simulink model "modele_ericc_correcteur"  (R2016b)
settings: Solver=VariableStepAuto  StartTime=0.0  StopTime=2.5  RelTol=1e-3
InitFcn:
  | ericc3_DataFile
values from neighbouring files (symbols this model uses):
  Cr = 0.01    [data_modele_ericc.m]
  fv = 1/8547    (= 0.000117000117)    [data_modele_ericc.m]
  Jeq = fv*0.178    (= 2.0826020826e-05)    [data_modele_ericc.m]
  KAN = 2*1e6/1080    (= 1851.85185185)    [data_modele_ericc.m]
  Kc = 2000/(2*pi)    (= 318.309886184)    [data_modele_ericc.m]
  Kd = 0    [data_modele_ericc.m]
  Ki = 2E5    (= 200000)    [data_modele_ericc.m]
  Kp = 1e6    (= 1000000)    [data_modele_ericc.m]
  Kr = 3/1000    (= 0.003)    [data_modele_ericc.m]
  Ks = Kc/(Kr*KAN)    (= 57.2957795131)    [data_modele_ericc.m]
  Kt = 0.043    [data_modele_ericc.m]
  Kv = 0.17    [data_modele_ericc.m]
settings Model: Creator=emiliendurif  LastModifiedBy=emiliendurif
settings SolverCC: ZeroCrossAlgorithm=Adaptive

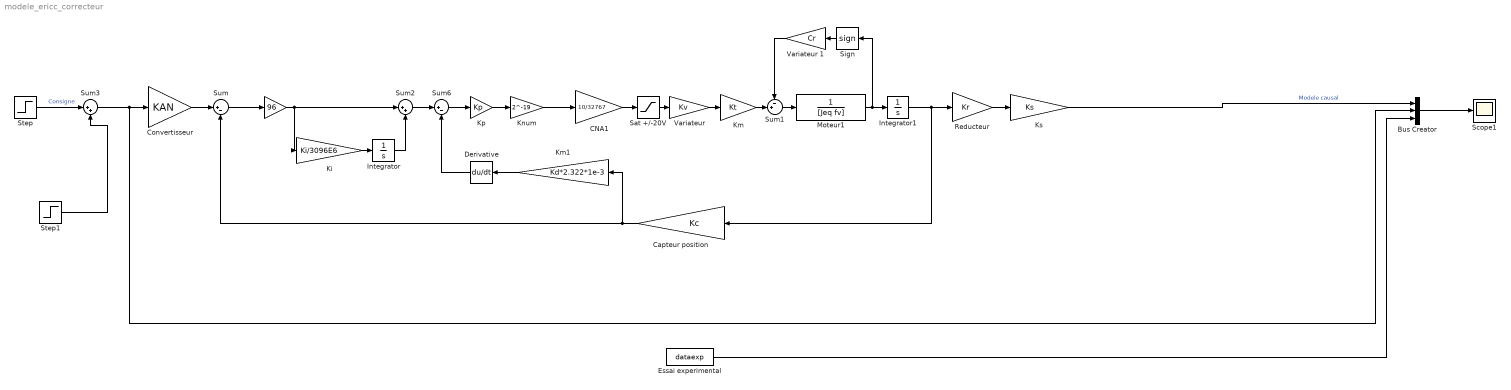
== system modele_ericc_correcteur ==
  " " : Gain  Gain=96
  Bus Creator : BusCreator  Inputs=3
  CNA1 : Gain  Gain=10/32767
  "Capteur position " : Gain  Gain=Kc
  Convertisseur : Gain  Gain=KAN
  Derivative : Derivative
  Essai experimental : FromWorkspace  VariableName=dataexp  OutDataTypeStr=fixdt('double', 'DataTypeOverride', 'Off')  SampleTime=0.007  OutputAfterFinalValue=Setting to zero
  Integrator : Integrator
  Integrator1 : Integrator
  Ki : Gain  Gain=Ki/3096E6
  Km : Gain  Gain=Kt
  Km1 : Gain  Gain=Kd*2.322*1e-3
  Knum : Gain  Gain=2^-19
  Kp : Gain  Gain=Kp
  Ks : Gain  Gain=Ks
  Moteur1 : TransferFcn  Denominator=[Jeq fv]
  Reducteur : Gain  Gain=Kr
  Sat +/-20V : Saturate  UpperLimit=10  LowerLimit=-10
  Scope1 : Scope
  Sign : Signum
  Step : Step  Time=0  After=30  SampleTime=0  ZeroCross=off
  Step1 : Step  Time=1.1  After=-30  SampleTime=0  ZeroCross=off
  Sum : Sum  Inputs=|+-
  Sum1 : Sum  Inputs=-+|
  Sum2 : Sum  Inputs=|++
  Sum3 : Sum  Inputs=|++
  Sum6 : Sum  Inputs=|+-
  "Variateur " : Gain  Gain=Kv
  Variateur 1 : Gain  Gain=Cr
  wires:
  Km/1 -> Sum1/2
  Step/1 -> Sum3/1  "Consigne"
  "Variateur "/1 -> Km/1
  Moteur1/1 -> Sign/1, Integrator1/1
  Integrator1/1 -> "Capteur position "/1, Reducteur/1
  Reducteur/1 -> Ks/1
  Ks/1 -> Bus Creator/1  "Modele causal"
  Bus Creator/1 -> Scope1/1
  Sum/1 -> " "/1
  " "/1 -> Ki/1, Sum2/1
  Integrator/1 -> Sum2/2
  Ki/1 -> Integrator/1
  Sum1/1 -> Moteur1/1
  Knum/1 -> CNA1/1
  "Capteur position "/1 -> Km1/1, Sum/2
  Kp/1 -> Knum/1
  Step1/1 -> Sum3/2
  Sign/1 -> Variateur 1/1
  Sum3/1 -> Convertisseur/1, Bus Creator/2
  Convertisseur/1 -> Sum/1
  Essai experimental/1 -> Bus Creator/3
  Sum6/1 -> Kp/1
  Sum2/1 -> Sum6/1
  Km1/1 -> Derivative/1
  Derivative/1 -> Sum6/2
  CNA1/1 -> Sat +/-20V/1
  Sat +/-20V/1 -> "Variateur "/1
  Variateur 1/1 -> Sum1/1
